simulink model "Parallel_R2015b"  (R2017a)
settings: Solver=ode4  StartTime=0  StopTime=1200  FixedStep=0.1  MaxStep=0.05  RelTol=1e-5
values from neighbouring files (symbols this model uses):
  Cd = 0.26    [Batch_vary_rated_power_initialise.m]    (also in Parallel_Initiate.m)
  Cr = 0.008    [Batch_vary_rated_power_initialise.m]    (also in Parallel_Initiate.m)
  Density = (85*19.6e6 + 15*32e6)/100    (= 21460000)    [Batch_vary_rated_power_initialise.m]    (also in Parallel_Initiate.m)
  Depletion = 0    [Batch_vary_rated_power_initialise.m]    (also in Parallel_Initiate.m)
  EtaEM = [Eta(length(w):-1:1,length(Tref):-1:1) Eta(length(w):-1:1,2:length(Tref)) ... (first row only)    [PMSM_plot_general_map.m]
  EtaICE = EtaICE_DIESEL    [Batch_vary_rated_power_initialise.m]    (also in Parallel_Initiate.m)
  EtaPE = 0.96    [Batch_vary_rated_power_initialise.m]    (also in Parallel_Initiate.m = 0.98)
  grav = 9.81    [Batch_vary_rated_power_initialise.m]    (also in Parallel_Initiate.m)
  Hybrid = 1    [Batch_vary_rated_power_initialise.m]    (also in Parallel_Initiate.m)
  ksoc = max(Wbatt)/400/Tau_charge    [Batch_vary_rated_power_initialise.m]    (also in Parallel_Initiate.m)
  Mv = 1325 + 250    (= 1575)    [Batch_vary_rated_power_initialise.m]    (also in Parallel_Initiate.m)
  Number_of_gears = 5    [Batch_vary_rated_power_initialise.m]    (also in Parallel_Initiate.m)
  OnOffMax = SOC_batt_ref - eps    [Batch_vary_rated_power_initialise.m]    (also in Parallel_Initiate.m)
  OnOffMin = 30    [Batch_vary_rated_power_initialise.m]    (also in Parallel_Initiate.m)
  Paux = 600    [Batch_vary_rated_power_initialise.m]    (also in Parallel_Initiate.m)
  Pem_max = EMpower*Hybrid+2000*(1-Hybrid)    [Batch_vary_rated_power_initialise.m]    (also in Parallel_Initiate.m = 50000)
  Pice_max = ICEpower*Hybrid+ICEconventional*(1-Hybrid)    [Batch_vary_rated_power_initialise.m]    (also in Parallel_Initiate.m = 65973)
  PtoT = zeros(length(P),4)    [CreateICEmap.m]
  rho_air = 1.225    [Batch_vary_rated_power_initialise.m]    (also in Parallel_Initiate.m)
  rw = 0.30    (= 0.3)    [Batch_vary_rated_power_initialise.m]    (also in Parallel_Initiate.m)
  SOC_batt_ref = 70    [Batch_vary_rated_power_initialise.m]    (also in Parallel_Initiate.m)
  StopAndGo = 0    [Batch_vary_rated_power_initialise.m]    (also in Parallel_Initiate.m)
  Tau_charge = 1    [Batch_vary_rated_power_initialise.m]    (also in Parallel_Initiate.m)
  Tem_max = TorqueEMmax*Hybrid+10*(1-Hybrid)    (= 200)    [Batch_vary_rated_power_initialise.m]    (also in Parallel_Initiate.m = 400)
  Tice_max = Pice_max/(wice_max*row/(length(EtaICE)-1))    [Batch_vary_rated_power_initialise.m]    (also in Parallel_Initiate.m)
  utvx_max = wice_max/((vmax/5)/rw)    (= 15.9043128088)    [Batch_vary_rated_power_initialise.m]    (also in Parallel_Initiate.m)
  Utvx_vect = zeros(1,Number_of_gears+1)    [Batch_vary_rated_power_initialise.m]    (also in Parallel_Initiate.m)
  Wbatt = 100*3600*13    (= 4680000)    [Batch_vary_rated_power_initialise.m]    (also in Parallel_Initiate.m)
  wice_max = 4500*2*pi/60    (= 471.238898038)    [Batch_vary_rated_power_initialise.m]    (also in Parallel_Initiate.m)
  wice_min = 700*2*pi/60    (= 73.3038285838)    [Batch_vary_rated_power_initialise.m]    (also in Parallel_Initiate.m = 83.7758040957)
undefined symbols (not defined in the file or in its folder): Av, EtaBATT, Pbatt, Pice_max_parallel, sfunxy, Tlim_ice, Wice
undefined symbols (not defined in the file): EMpower, FuelConsICE, ICEpower, Tem, Tice, utvx_min, vmax, Wem
libraries: simulink_need_slupdate x1
(part 2 of 2)

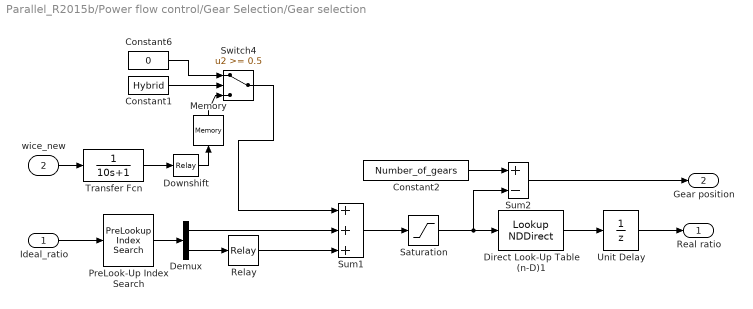
== system Parallel_R2015b/Power flow control/Gear Selection/Gear selection ==
  Ideal_ratio : Inport
  wice_new : Inport  Port=2
  Constant1 : Constant  Value=Hybrid
  Constant2 : Constant  Value=Number_of_gears
  Constant6 : Constant  Value=0
  Demux : Demux  Outputs=2
  Direct Look-Up Table (n-D)1 : LookupNDDirect  NumberOfTableDimensions=1  Table=Utvx_vect
  Downshift : Relay  OnSwitchValue=0.85*wice_max  OffSwitchValue=0.40*wice_max  OnOutputValue=0  OffOutputValue=Speedy
  Memory : Memory
  PreLook-Up Index Search : simulink_need_slupdate/PreLookup Index Search  bpData=Utvx_vect  searchMode=Binary Search  cacheBpFlag=off  outputFlag=off  IndexDataType=uint32  extrapMode=Linear Extrapolation  rangeErrorMode=None
      settings: SourceProductName=Simulink  SourceProductBaseCode=SL
  Relay : Relay  OnSwitchValue=0.55  OffSwitchValue=0.45
  Saturation : Saturate  UpperLimit=Number_of_gears-1  LowerLimit=0
  Sum1 : Sum  Inputs=+++  SaturateOnIntegerOverflow=on
  Sum2 : Sum  Inputs=+-  SaturateOnIntegerOverflow=on
  Switch4 : Switch  Threshold=0.5  SaturateOnIntegerOverflow=on  InputSameDT=on
  Transfer Fcn : TransferFcn  Denominator=[10 1]
  Unit Delay : UnitDelay  InitialCondition=utvx_max
  Real ratio : Outport
  Gear position : Outport  Port=2
  wires:
  Ideal_ratio/1 -> PreLook-Up Index Search/1
  Constant1/1 -> Switch4/2
  Switch4/1 -> Sum1/1
  wice_new/1 -> Transfer Fcn/1
  Downshift/1 -> Memory/1
  Transfer Fcn/1 -> Downshift/1
  Memory/1 -> Switch4/3
  Constant6/1 -> Switch4/1
  PreLook-Up Index Search/1 -> Demux/1
  Demux/2 -> Relay/1
  Sum1/1 -> Saturation/1
  Relay/1 -> Sum1/3
  Demux/1 -> Sum1/2
  Direct Look-Up Table (n-D)1/1 -> Unit Delay/1
  Constant2/1 -> Sum2/1
  Sum2/1 -> Gear position/1
  Unit Delay/1 -> Real ratio/1
  Saturation/1 -> Sum2/2, Direct Look-Up Table (n-D)1/1

== system Parallel_R2015b/Power flow control/Optimal operating point/LP-filter ==
  P ice* : Inport
  Gain2 : Gain  Gain=1/(Tau_charge)  SaturateOnIntegerOverflow=on  OutDataTypeStr=Inherit: Same as input  ParamDataTypeStr=Inherit: Same as input
  Sum3 : Sum  Inputs=+-  SaturateOnIntegerOverflow=on  InputSameDT=on  OutDataTypeStr=Inherit: Same as first input
  Wbatt : Integrator  UpperSaturationLimit=Pice_max_parallel  LowerSaturationLimit=0
  P ice : Outport  InitialOutput=0
  wires:
  P ice*/1 -> Sum3/1
  Sum3/1 -> Gain2/1
  Gain2/1 -> Wbatt/1
  Wbatt/1 -> Sum3/2, P ice/1
